simulink model "FlatBeam_force"  (R2019a)
settings: Solver=VariableStepAuto  StartTime=0.0  StopTime=simtime  FixedStep=step_size  RelTol=1e-7  EnableMultiTasking=on
values from neighbouring files (symbols this model uses):
  A = [zeros(n,n), eye(n) ... (first row only)    [ClampedBeam_simulink.m]    (also in ClampedClampedBeam_NMA.m; FaltBeam_NMA.m)
  a = 0.02*2*pi    (= 0.125663706144)    [ClampedBeam_simulink.m]    (also in ClampedClampedBeam_NMA.m; FaltBeam_NMA.m)
  B = [zeros(n,1);oscillator.M\loc_exc]    [ClampedBeam_simulink.m]    (also in ClampedClampedBeam_NMA.m; FaltBeam_NMA.m = zeros(2*n,2*n))
  B_nl = [zeros(n,1);oscillator.M\loc_nl]    [ClampedBeam_simulink.m]    (also in ClampedClampedBeam_NMA.m = [zeros(n,1);oscillator.M\loc_nl]*NL_coeff; FaltBeam_NMA.m = B)
  I = 50    [ClampedBeam_simulink.m]    (also in ClampedClampedBeam_NMA.m; FaltBeam_NMA.m)
  NL_coeff = oscillator.nonlinear_elements{1}.coefficients    [ClampedBeam_simulink.m]    (also in ClampedClampedBeam_NMA.m)
  omega_0 = OM2    [ClampedBeam_simulink.m]    (also in ClampedClampedBeam_NMA.m = om_lin; FaltBeam_NMA.m = om_lin(imod))
  P = 5    [ClampedBeam_simulink.m]    (also in ClampedClampedBeam_NMA.m = 10; FaltBeam_NMA.m)
  phase_lag = 90    [ClampedBeam_simulink.m]    (also in ClampedClampedBeam_NMA.m; FaltBeam_NMA.m)
  T_disp = [eye(n,n) zeros(n,n)]    [ClampedBeam_simulink.m]    (also in ClampedClampedBeam_NMA.m = [eye(n,n) zeros(n,n)]*PHI_L_2; FaltBeam_NMA.m)
  T_exc = zeros(1,2*n)    [ClampedBeam_simulink.m]    (also in ClampedClampedBeam_NMA.m; FaltBeam_NMA.m)
  T_nl = zeros(1,2*n)    [ClampedBeam_simulink.m]    (also in ClampedClampedBeam_NMA.m; FaltBeam_NMA.m)
  x0beam = 0    [ClampedBeam_simulink.m]    (also in ClampedClampedBeam_NMA.m; FaltBeam_NMA.m)
  x0vco = 0    [ClampedBeam_simulink.m]    (also in ClampedClampedBeam_NMA.m; FaltBeam_NMA.m)
libraries: simulink x1
settings Model: SimulationMode=accelerator  Creator=peter  LastModifiedBy=eve_lian
settings SolverCC: ZeroCrossAlgorithm=Adaptive  SolverResetMethod=Robust
settings DataIOCC: LimitDataPoints=on  SaveFormat=Array  SignalLoggingSaveFormat=ModelDataLogs  ReturnWorkspaceOutputs=off
settings OptimizationCC: LifeSpan=inf
settings DebuggingCC: UnderspecifiedInitializationDetection=Classic  MergeDetectMultiDrivingBlocksExec=none  SolverPrmCheckMsg=warning  MultiTaskDSMMsg=warning  MultiTaskCondExecSysMsg=none  StateNameClashWarn=warning  SFUnexpectedBacktrackingDiag=warning  SFNoUnconditionalDefaultTransitionDiag=warning  SFExecutionAtInitializationDiag=none  ArithmeticOperatorsInVariantConditions=warning
settings HardwareCC: ProdBitPerPointer=32  ProdBitPerSizeT=32  ProdBitPerPtrDiffT=32  ProdLargestAtomicFloat=None  ProdIntDivRoundTo=Undefined  ProdEndianess=Unspecified  ProdWordSize=32  ProdHWDeviceType=32-bit Generic
settings ModelReferenceCC: UpdateModelReferenceTargets=IfOutOfDate  PropagateSignalLabelsOutOfModel=off
settings SFSimCC: SFSimEcho=off  SimUseLocalCustomCode=off
settings RTWCC: RTWUseLocalCustomCode=off
settings CodeAppCC: StateflowObjectComments=on
settings GRTTargetCC: TargetLangStandard=C89/C90 (ANSI)  GeneratePreprocessorConditionals=Disable all
settings ConfigComp: CovMetricSettings=dw  CovHtmlReporting=on  CovSaveCumulativeToWorkspaceVar=on  CovSaveSingleToWorkspaceVar=on  CovExternalEMLEnable=off
settings SimscapeCC: SimscapeNormalizeSystem=off

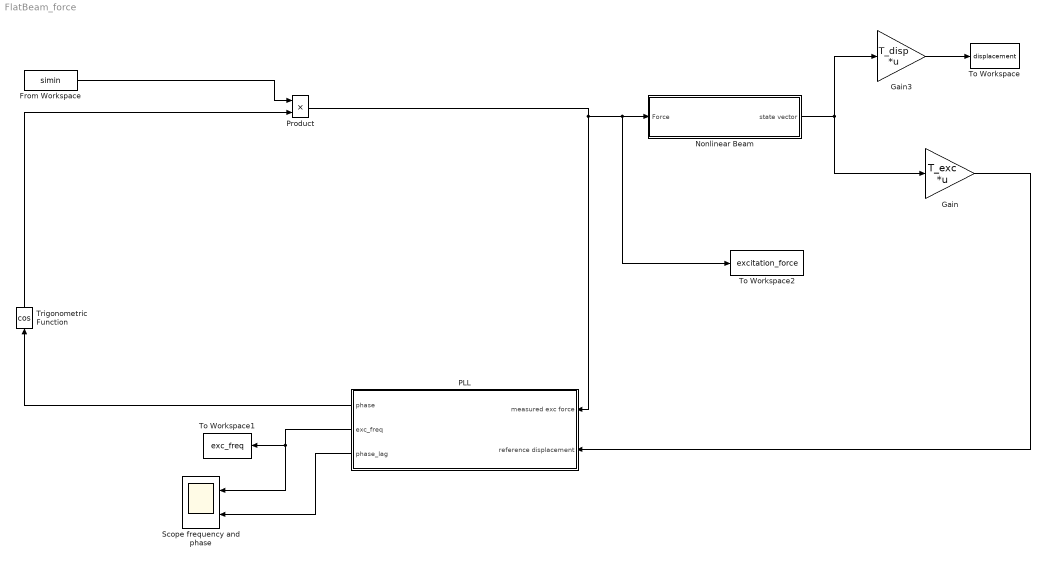
== system FlatBeam_force ==
  From Workspace : FromWorkspace  VariableName=simin  SampleTime=0
  Gain : Gain  Gain=T_exc  Multiplication=Matrix(K*u)
  Gain3 : Gain  Gain=T_disp  Multiplication=Matrix(K*u)
  Nonlinear Beam : Subsystem
  PLL : Subsystem
  Product : Product  RndMeth=Zero
  Scope frequency and phase : Scope  NumInputPorts=2
  To Workspace : ToWorkspace  VariableName=displacement  SaveFormat=Structure With Time  SampleTime=-1
  To Workspace1 : ToWorkspace  VariableName=exc_freq  SaveFormat=Structure With Time  SampleTime=-1
  To Workspace2 : ToWorkspace  VariableName=excitation_force  SaveFormat=Structure With Time  SampleTime=-1
  Trigonometric Function : Trigonometry  Operator=cos
  wires:
  Nonlinear Beam/1(state vector) -> Gain3/1, Gain/1
  Gain/1 -> PLL/2(reference displacement)
  Trigonometric Function/1 -> Product/2
  Product/1 -> To Workspace2/1, Nonlinear Beam/1(Force), PLL/1(measured exc force)
  From Workspace/1 -> Product/1
  PLL/1(phase) -> Trigonometric Function/1
  Gain3/1 -> To Workspace/1
  PLL/3(phase_lag) -> Scope frequency and phase/2
  PLL/2(exc_freq) -> To Workspace1/1, Scope frequency and phase/1

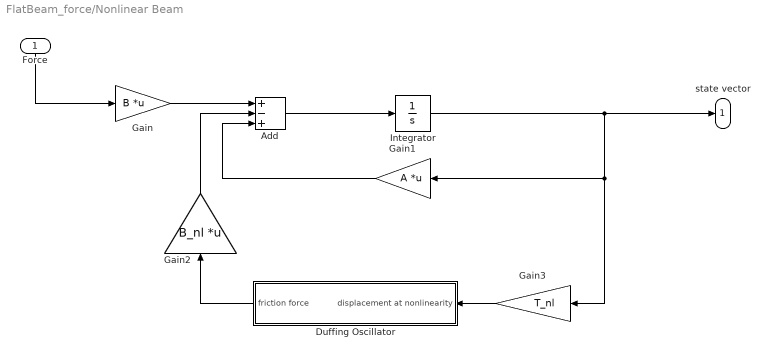
== system FlatBeam_force/Nonlinear Beam ==
  Force : Inport
  Add : Sum  Inputs=+-+
  Duffing Oscillator : Subsystem
  Gain : Gain  Gain=B  Multiplication=Matrix(K*u) (u vector)
  Gain1 : Gain  Gain=A  Multiplication=Matrix(K*u) (u vector)
  Gain2 : Gain  Gain=B_nl  Multiplication=Matrix(K*u) (u vector)
  Gain3 : Gain  Gain=T_nl
  Integrator : Integrator  InitialCondition=x0beam
  state vector : Outport
  wires:
  Force/1 -> Gain/1
  Gain/1 -> Add/1
  Add/1 -> Integrator/1
  Integrator/1 -> Gain3/1, Gain1/1, state vector/1
  Gain1/1 -> Add/3
  Gain2/1 -> Add/2
  Duffing Oscillator/1(friction force) -> Gain2/1
  Gain3/1 -> Duffing Oscillator/1(displacement at nonlinearity)

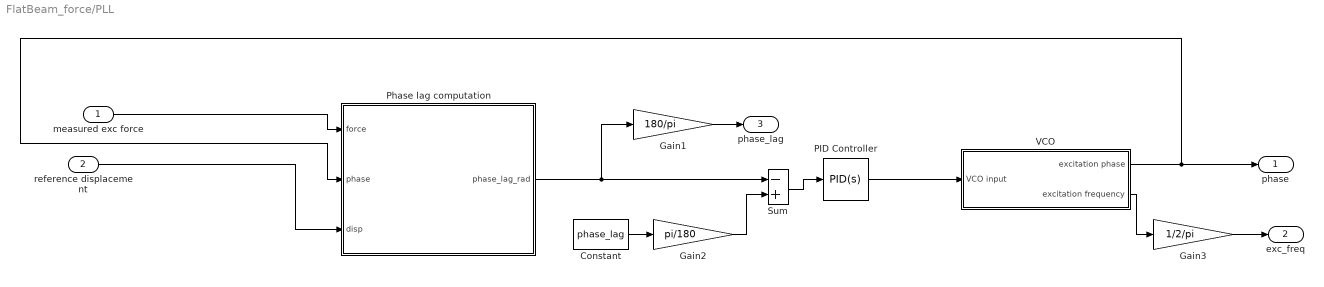
== system FlatBeam_force/PLL ==
  measured exc force : Inport
  reference displacement : Inport  Port=2
  Constant : Constant  Value=phase_lag
  Gain1 : Gain  Gain=180/pi
  Gain2 : Gain  Gain=pi/180
  Gain3 : Gain  Gain=1/2/pi
  PID Controller : simulink/Continuous/PID Controller  Controller=PID  Form=Parallel  TimeDomain=Continuous-time  SampleTime=-1  IntegratorMethod=Forward Euler  FilterMethod=Forward Euler  ControllerParametersSource=internal  P=P  I=I  D=0  UseFilter=on  N=100  TunerSelectOption=Transfer Function Based (PID Tuner App)  InitialConditionSource=internal  InitialConditionForIntegrator=0  InitialConditionForFilter=0  DifferentiatorICPrevScaledInput=0  ExternalReset=none  IgnoreLimit=on  TrackingMode=off  Kt=1  LimitOutput=off  UpperSaturationLimit=inf  LowerSaturationLimit=-inf  LinearizeAsGain=on  AntiWindupMode=none  Kb=1  POutMin=[]  POutMax=[]  IOutMin=[]  IOutMax=[]  DOutMin=[]  DOutMax=[]  NOutMin=[]  NOutMax=[]  SumOutMin=[]  SumOutMax=[]  SaturationOutMin=[]  SaturationOutMax=[]  PParamMin=[]  PParamMax=[]  IParamMin=[]  IParamMax=[]  DParamMin=[]  DParamMax=[]  NParamMin=[]  NParamMax=[]  KbParamMin=[]  KbParamMax=[]  KtParamMin=[]  KtParamMax=[]  KbOutMin=[]  KbOutMax=[]  KtOutMin=[]  KtOutMax=[]  IntegratorOutMin=[]  IntegratorOutMax=[]  FilterOutMin=[]  FilterOutMax=[]  SumI1OutMin=[]  SumI1OutMax=[]  SumI2OutMin=[]  SumI2OutMax=[]  SumI3OutMin=[]  SumI3OutMax=[]  SumI4OutMin=[]  SumI4OutMax=[]  SumDOutMin=[]  SumDOutMax=[]  DifferentiatorOutMin=[]  DifferentiatorOutMax=[]  FilterDiffOutCoefMin=[]  FilterDiffOutCoefMax=[]  ReciprocalOutMin=[]  ReciprocalOutMax=[]  SumDenOutMin=[]  SumDenOutMax=[]  SumNumOutMin=[]  SumNumOutMax=[]  DivideOutMin=[]  DivideOutMax=[]  IntegratorContinuousStateAttributes=''  IntegratorStateMustResolveToSignalObject=off  IntegratorRTWStateStorageClass=Auto  FilterContinuousStateAttributes=''  FilterStateMustResolveToSignalObject=off  FilterRTWStateStorageClass=Auto  ParallelPVariant=InternalParameters  IdealPVariant=Disabled  IVariant=InternalParameters  DVariant=InternalParameters  IntegratorVariant=Continuous  SatVariant=Disabled  AWVariant=Passthrough  PCopyVariant=Disabled  TRVariant=Disabled  FdbkBlocksVariant=Forward  IdealPFdbkVariant=Disabled  SatFdbkVariant=Disabled  DerivativeFilterVariant=ContFilter  NVariant=InternalParameters  NCopyVariant=Disabled  FilterICVariant=InternalICsFilter  IntegratorICVariant=InternalICs  ExternalResetVariant=Disabled  TRSumVariant=Passthrough  SumFdbkVariant=Disabled  SumVariant=Sum_PID
  Phase lag computation : Subsystem
  Sum : Sum  Inputs=-+
  VCO : Subsystem
  phase : Outport
  exc_freq : Outport  Port=2
  phase_lag : Outport  Port=3
  wires:
  VCO/1(excitation phase) -> phase/1, Phase lag computation/2(phase)
  PID Controller/1 -> VCO/1(VCO input)
  reference displacement/1 -> Phase lag computation/3(disp)
  measured exc force/1 -> Phase lag computation/1(force)
  Phase lag computation/1(phase_lag_rad) -> Gain1/1, Sum/1
  VCO/2(excitation frequency) -> Gain3/1
  Constant/1 -> Gain2/1
  Sum/1 -> PID Controller/1
  Gain2/1 -> Sum/2
  Gain3/1 -> exc_freq/1
  Gain1/1 -> phase_lag/1

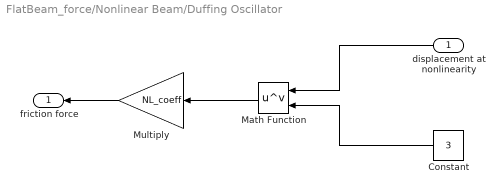
== system FlatBeam_force/Nonlinear Beam/Duffing Oscillator ==
  displacement at nonlinearity : Inport
  Constant : Constant  Value=3
  Math Function : Math  Operator=pow  SaturateOnIntegerOverflow=on
  Multiply : Gain  Gain=NL_coeff
  friction force : Outport
  wires:
  Math Function/1 -> Multiply/1
  displacement at nonlinearity/1 -> Math Function/1
  Constant/1 -> Math Function/2
  Multiply/1 -> friction force/1

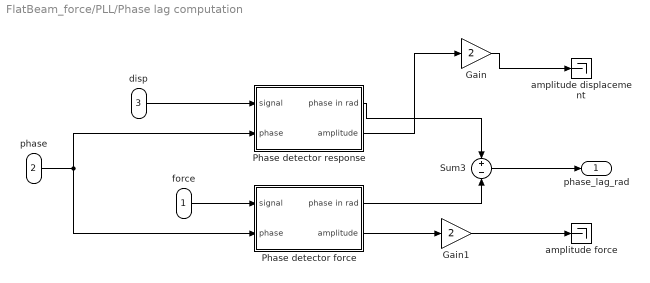
== system FlatBeam_force/PLL/Phase lag computation ==
  force : Inport
  phase : Inport  Port=2
  disp : Inport  Port=3
  Gain : Gain  Gain=2
  Gain1 : Gain  Gain=2
  Phase detector force : Subsystem
  Phase detector response : Subsystem
  Sum3 : Sum  Inputs=+-
  amplitude displacement : Terminator
  amplitude force : Terminator
  phase_lag_rad : Outport
  wires:
  Phase detector response/1(phase in rad) -> Sum3/1
  Sum3/1 -> phase_lag_rad/1
  Phase detector force/1(phase in rad) -> Sum3/2
  phase/1 -> Phase detector force/2(phase), Phase detector response/2(phase)
  disp/1 -> Phase detector response/1(signal)
  force/1 -> Phase detector force/1(signal)
  Phase detector response/2(amplitude) -> Gain/1
  Phase detector force/2(amplitude) -> Gain1/1
  Gain1/1 -> amplitude force/1
  Gain/1 -> amplitude displacement/1

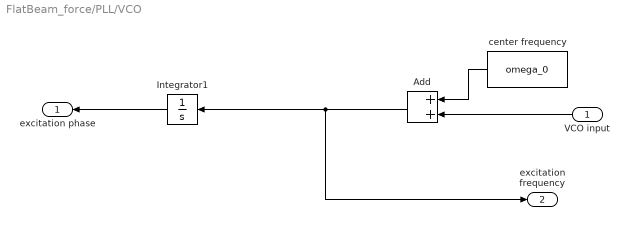
== system FlatBeam_force/PLL/VCO ==
  VCO input : Inport
  Add : Sum
  Integrator1 : Integrator  InitialCondition=x0vco
  center frequency : Constant  Value=omega_0
  excitation phase : Outport
  excitation frequency : Outport  Port=2
  wires:
  VCO input/1 -> Add/2
  center frequency/1 -> Add/1
  Integrator1/1 -> excitation phase/1
  Add/1 -> excitation frequency/1, Integrator1/1

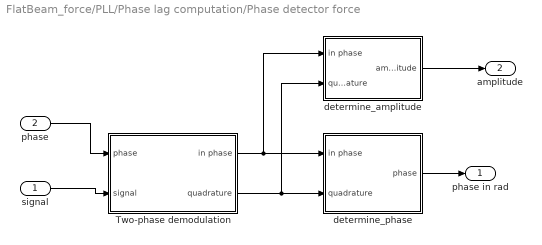
== system FlatBeam_force/PLL/Phase lag computation/Phase detector force ==
  signal : Inport
  phase : Inport  Port=2
  Two-phase demodulation : Subsystem
  determine_amplitude : Subsystem
  determine_phase : Subsystem
  phase in rad : Outport
  amplitude : Outport  Port=2
  wires:
  phase/1 -> Two-phase demodulation/1(phase)
  signal/1 -> Two-phase demodulation/2(signal)
  Two-phase demodulation/2(quadrature) -> determine_amplitude/2(quadrature), determine_phase/2(quadrature)
  determine_phase/1(phase) -> phase in rad/1
  Two-phase demodulation/1(in phase) -> determine_amplitude/1(in phase), determine_phase/1(in phase)
  determine_amplitude/1(amplitude) -> amplitude/1

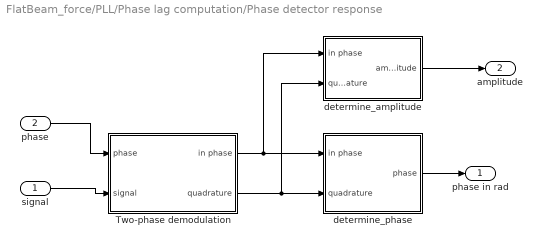
== system FlatBeam_force/PLL/Phase lag computation/Phase detector response ==
  signal : Inport
  phase : Inport  Port=2
  Two-phase demodulation : Subsystem
  determine_amplitude : Subsystem
  determine_phase : Subsystem
  phase in rad : Outport
  amplitude : Outport  Port=2
  wires:
  phase/1 -> Two-phase demodulation/1(phase)
  signal/1 -> Two-phase demodulation/2(signal)
  Two-phase demodulation/2(quadrature) -> determine_amplitude/2(quadrature), determine_phase/2(quadrature)
  determine_phase/1(phase) -> phase in rad/1
  Two-phase demodulation/1(in phase) -> determine_amplitude/1(in phase), determine_phase/1(in phase)
  determine_amplitude/1(amplitude) -> amplitude/1

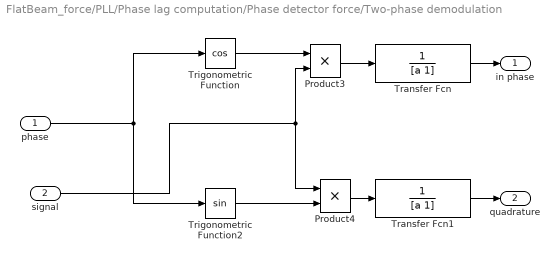
== system FlatBeam_force/PLL/Phase lag computation/Phase detector force/Two-phase demodulation ==
  phase : Inport
  signal : Inport  Port=2
  Product3 : Product
  Product4 : Product
  Transfer Fcn : TransferFcn  Denominator=[a 1]
  Transfer Fcn1 : TransferFcn  Denominator=[a 1]
  Trigonometric Function : Trigonometry  Operator=cos
  Trigonometric Function2 : Trigonometry
  in phase : Outport
  quadrature : Outport  Port=2
  wires:
  Trigonometric Function2/1 -> Product4/2
  signal/1 -> Product3/2, Product4/1
  phase/1 -> Trigonometric Function/1, Trigonometric Function2/1
  Trigonometric Function/1 -> Product3/1
  Product3/1 -> Transfer Fcn/1
  Transfer Fcn1/1 -> quadrature/1
  Transfer Fcn/1 -> in phase/1
  Product4/1 -> Transfer Fcn1/1

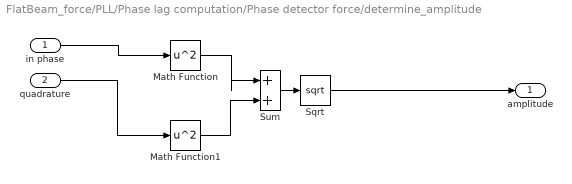
== system FlatBeam_force/PLL/Phase lag computation/Phase detector force/determine_amplitude ==
  in phase : Inport
  quadrature : Inport  Port=2
  Math Function : Math  Operator=square  SaturateOnIntegerOverflow=on
  Math Function1 : Math  Operator=square  SaturateOnIntegerOverflow=on
  Sqrt : Sqrt  SaturateOnIntegerOverflow=on
  Sum : Sum  Inputs=|++
  amplitude : Outport
  wires:
  Sqrt/1 -> amplitude/1
  quadrature/1 -> Math Function1/1
  in phase/1 -> Math Function/1
  Math Function/1 -> Sum/1
  Math Function1/1 -> Sum/2
  Sum/1 -> Sqrt/1

== system FlatBeam_force/PLL/Phase lag computation/Phase detector force/determine_phase ==
  in phase : Inport
  quadrature : Inport  Port=2
  Trigonometric Function1 : Trigonometry  Operator=atan2
  phase : Outport
  wires:
  Trigonometric Function1/1 -> phase/1
  in phase/1 -> Trigonometric Function1/2
  quadrature/1 -> Trigonometric Function1/1

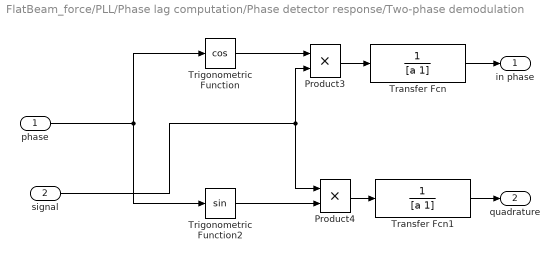
== system FlatBeam_force/PLL/Phase lag computation/Phase detector response/Two-phase demodulation ==
  phase : Inport
  signal : Inport  Port=2
  Product3 : Product
  Product4 : Product
  Transfer Fcn : TransferFcn  Denominator=[a 1]
  Transfer Fcn1 : TransferFcn  Denominator=[a 1]
  Trigonometric Function : Trigonometry  Operator=cos
  Trigonometric Function2 : Trigonometry
  in phase : Outport
  quadrature : Outport  Port=2
  wires:
  Trigonometric Function2/1 -> Product4/2
  signal/1 -> Product3/2, Product4/1
  phase/1 -> Trigonometric Function/1, Trigonometric Function2/1
  Trigonometric Function/1 -> Product3/1
  Product3/1 -> Transfer Fcn/1
  Transfer Fcn1/1 -> quadrature/1
  Transfer Fcn/1 -> in phase/1
  Product4/1 -> Transfer Fcn1/1

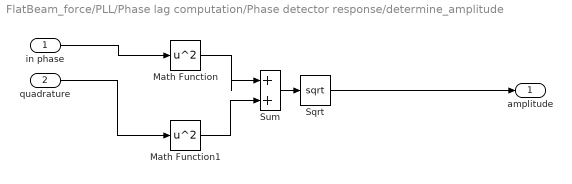
== system FlatBeam_force/PLL/Phase lag computation/Phase detector response/determine_amplitude ==
  in phase : Inport
  quadrature : Inport  Port=2
  Math Function : Math  Operator=square  SaturateOnIntegerOverflow=on
  Math Function1 : Math  Operator=square  SaturateOnIntegerOverflow=on
  Sqrt : Sqrt  SaturateOnIntegerOverflow=on
  Sum : Sum  Inputs=|++
  amplitude : Outport
  wires:
  Sqrt/1 -> amplitude/1
  quadrature/1 -> Math Function1/1
  in phase/1 -> Math Function/1
  Math Function/1 -> Sum/1
  Math Function1/1 -> Sum/2
  Sum/1 -> Sqrt/1

== system FlatBeam_force/PLL/Phase lag computation/Phase detector response/determine_phase ==
  in phase : Inport
  quadrature : Inport  Port=2
  Trigonometric Function1 : Trigonometry  Operator=atan2
  phase : Outport
  wires:
  Trigonometric Function1/1 -> phase/1
  in phase/1 -> Trigonometric Function1/2
  quadrature/1 -> Trigonometric Function1/1
